simulink model "QEI_Polling"  (R2024b)
settings: Solver=FixedStepAuto  StartTime=0.0  StopTime=inf  FixedStep=0.001  RelTol=1e-3  EnableMultiTasking=on
libraries: stm32f4xxblockslib x5, stm32g4xxblockslib x3
settings Model: STM32="{\"DigitalPortRead\":[{\"ID\":\"untitled1:6\"},{\"ID\":\"untitled1:7\"},{\"ID\":\"untitled1:8\"},{\"ID\":\"untitled1:9\"},{\"ID\":\"untitled1:10\"},{\"ID\":\"QEI_Polling:10\"},{\"ID\":\"QEI_Polling:9\"},{\"ID\":\"QEI_Polling:8\"},{\"ID\":\"QEI_Polling:7\"},{\"ID\":\"QEI_Polling:6\"}],\"EncoderBlockForG4\":[{\"ID\":\"untitled1:29\"},{\"ID\":\"untitled1:30\"},{\"ID\":\"untitled1:31\"},{\"ID\":\"QEI_Polling:29\"},{\"ID\":\"QEI_Polling:30\"},{\"ID\":\"QEI_Polling:31\"}]}"  Creator=spwkp  LastModifiedBy=spwkp
settings OptimizationCC: DefaultParameterBehavior=Inlined  EnhancedBackFolding=on  PassReuseOutputArgsAs=Individual arguments  ZeroExternalMemoryAtStartup=off  ZeroInternalMemoryAtStartup=off  MaxStackSize=512  OptimizeBlockOrder=speed  DifferentSizesBufferReuse=on  OptimizationCustomize=off  EfficientTunableParamExpr=on
settings DebuggingCC: ParameterTunabilityLossMsg=error
settings HardwareCC: ProdBitPerPointer=32  ProdBitPerSizeT=32  ProdBitPerPtrDiffT=32  ProdLargestAtomicInteger=Long  ProdLargestAtomicFloat=Double  ProdWordSize=32  ProdLongLongMode=on  ProdHWDeviceType=ARM Compatible->ARM Cortex-M
settings SFSimCC: MATLABDynamicMemAlloc=off
settings RTWCC: Description=Embedded Coder  SystemTargetFile=ert.tlc  HardwareBoard=STM32G4xx Based  TemplateMakefile=ert_default_tmf  Toolchain=GNU Tools for ARM Embedded Processors
settings CodeAppCC: ForceParamTrailComments=on  IgnoreCustomStorageClasses=off  OperatorAnnotations=on  SimulinkDataObjDesc=on  SFDataObjDesc=on  InsertBlockDesc=on
settings ERTTargetCC: TargetLangStandard=C99 (ISO)  CodeReplacementLibrary=ARM Cortex-M  ExtModeTransport=3  ExtModeStaticAlloc=on  ExtModeStaticAllocSize=2048  ExtModeMexFile=ext_xcp  ExtModeIntrfLevel=Level2 - Open

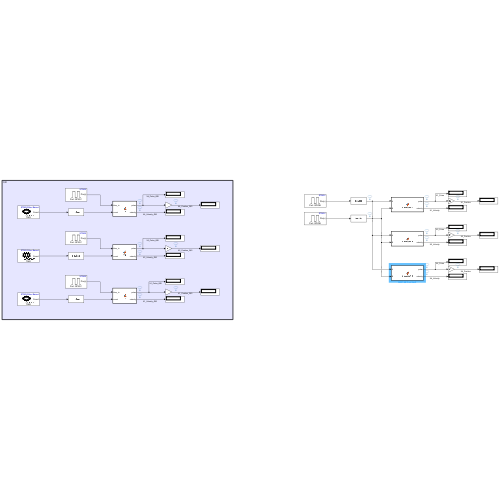
[thumbnail: Simulink's stored preview of the top-level diagram]
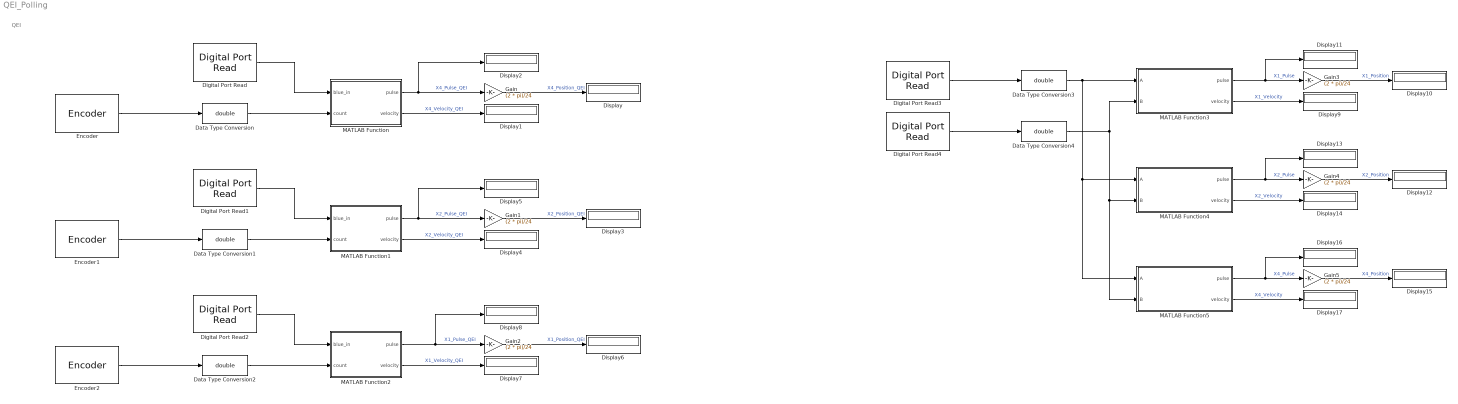
== system QEI_Polling ==
  note: QEI
  Data Type Conversion{,1..4} (5 alike) : DataTypeConversion  OutDataTypeStr=double  SaturateOnIntegerOverflow=off  RndMeth=Floor
  Digital Port Read : stm32f4xxblockslib/Digital Port Read  PortName=GPIOC  PinNumber=[13]  ReadOperation=on  IOAsArray=on  SampleTime=-1  EnableSimPort=off  hoistedMaskSrc=ECSoC/ECSimCodegen/Digital Port Read
      settings: LibrarySourceBlock=stm32g4xxblockslib/Digital Port Read
  Digital Port Read1 : stm32f4xxblockslib/Digital Port Read  PortName=GPIOC  PinNumber=[13]  ReadOperation=on  IOAsArray=on  SampleTime=-1  EnableSimPort=off  hoistedMaskSrc=ECSoC/ECSimCodegen/Digital Port Read
      settings: LibrarySourceBlock=stm32g4xxblockslib/Digital Port Read
  Digital Port Read2 : stm32f4xxblockslib/Digital Port Read  PortName=GPIOC  PinNumber=[13]  ReadOperation=on  IOAsArray=on  SampleTime=-1  EnableSimPort=off  hoistedMaskSrc=ECSoC/ECSimCodegen/Digital Port Read
      settings: LibrarySourceBlock=stm32g4xxblockslib/Digital Port Read
  Digital Port Read3 : stm32f4xxblockslib/Digital Port Read  PortName=GPIOB  PinNumber=[5]  ReadOperation=on  IOAsArray=on  SampleTime=-1  EnableSimPort=off  hoistedMaskSrc=ECSoC/ECSimCodegen/Digital Port Read
      settings: LibrarySourceBlock=stm32g4xxblockslib/Digital Port Read
  Digital Port Read4 : stm32f4xxblockslib/Digital Port Read  PortName=GPIOB  PinNumber=[4]  ReadOperation=on  IOAsArray=on  SampleTime=-1  EnableSimPort=off  hoistedMaskSrc=ECSoC/ECSimCodegen/Digital Port Read
      settings: LibrarySourceBlock=stm32g4xxblockslib/Digital Port Read
  Display{,1..17} (18 alike) : Display
  Encoder : stm32g4xxblockslib/Encoder  TimerModule=TIM3  EnableResetInput=off  OutputCountAfterFirstIndex=off  OutputValidIndex=off  OutputDirection=off  OutputStatus=off  SampleTime=-1
  Encoder1 : stm32g4xxblockslib/Encoder  TimerModule=TIM4  EnableResetInput=off  OutputCountAfterFirstIndex=off  OutputValidIndex=off  OutputDirection=off  OutputStatus=off  SampleTime=-1
  Encoder2 : stm32g4xxblockslib/Encoder  TimerModule=TIM8  EnableResetInput=off  OutputCountAfterFirstIndex=off  OutputValidIndex=off  OutputDirection=off  OutputStatus=off  SampleTime=-1
  Gain{,1..5} (6 alike) : Gain  Gain=(2 * pi)/24
  MATLAB Function : MATLAB Function  TreatAsAtomicUnit=on
  MATLAB Function1 : MATLAB Function  TreatAsAtomicUnit=on
  MATLAB Function2 : MATLAB Function  TreatAsAtomicUnit=on
  MATLAB Function3 : MATLAB Function  TreatAsAtomicUnit=on
  MATLAB Function4 : MATLAB Function  TreatAsAtomicUnit=on
  MATLAB Function5 : MATLAB Function  TreatAsAtomicUnit=on
  wires:
  Data Type Conversion/1 -> MATLAB Function/2(count)
  Encoder1/1 -> Data Type Conversion1/1
  Gain3/1 -> Display10/1  "X1_Position"
  MATLAB Function2/2(velocity) -> Display7/1  "X1_Velocity_QEI"
  MATLAB Function3/2(velocity) -> Display9/1  "X1_Velocity"
  Data Type Conversion3/1 -> MATLAB Function4/1(A), MATLAB Function5/1(A), MATLAB Function3/1(A)
  Data Type Conversion2/1 -> MATLAB Function2/2(count)
  MATLAB Function3/1(pulse) -> Display11/1, Gain3/1  "X1_Pulse"
  Digital Port Read1/1 -> MATLAB Function1/1(blue_in)
  Encoder2/1 -> Data Type Conversion2/1
  Digital Port Read/1 -> MATLAB Function/1(blue_in)
  Digital Port Read4/1 -> Data Type Conversion4/1
  MATLAB Function5/1(pulse) -> Display16/1, Gain5/1  "X4_Pulse"
  MATLAB Function/1(pulse) -> Display2/1, Gain/1  "X4_Pulse_QEI"
  Gain5/1 -> Display15/1  "X4_Position"
  Data Type Conversion1/1 -> MATLAB Function1/2(count)
  MATLAB Function1/2(velocity) -> Display4/1  "X2_Velocity_QEI"
  Data Type Conversion4/1 -> MATLAB Function4/2(B), MATLAB Function5/2(B), MATLAB Function3/2(B)
  Gain1/1 -> Display3/1  "X2_Position_QEI"
  Digital Port Read3/1 -> Data Type Conversion3/1
  MATLAB Function4/1(pulse) -> Display13/1, Gain4/1  "X2_Pulse"
  Encoder/1 -> Data Type Conversion/1
  Digital Port Read2/1 -> MATLAB Function2/1(blue_in)
  MATLAB Function5/2(velocity) -> Display17/1  "X4_Velocity"
  MATLAB Function1/1(pulse) -> Display5/1, Gain1/1  "X2_Pulse_QEI"
  Gain/1 -> Display/1  "X4_Position_QEI"
  MATLAB Function/2(velocity) -> Display1/1  "X4_Velocity_QEI"
  Gain4/1 -> Display12/1  "X2_Position"
  Gain2/1 -> Display6/1  "X1_Position_QEI"
  MATLAB Function4/2(velocity) -> Display14/1  "X2_Velocity"
  MATLAB Function2/1(pulse) -> Display8/1, Gain2/1  "X1_Pulse_QEI"

== matlab function QEI_Polling/MATLAB Function1 ==
  data: blue_in input; pulse output; count input; velocity output
function [pulse, velocity] = X4(blue_in, count)
    %#codegen
    
    % ประกาศตัวแปร persistent เพื่อเก็บค่าตัวนับก่อนหน้าและตำแหน่งที่คลายห่อก่อนหน้า
    persistent previousCount unwrappedPositionPrev;
    
    % กำหนดค่าเริ่มต้นให้ตัวแปร persistent เมื่อเรียกใช้งานครั้งแรก
    if isempty(previousCount)
        previousCount = count;
        unwrappedPositionPrev = 0;  % กำหนดตำแหน่งคลายห่อเริ่มต้นเป็นศูนย์
    end

    % กำหนดขอบเขตของ encoder
    encoderMax = 65520;   % ค่าสูงสุดสำหรับ encoder แบบ 16-bit (0-65535)
    threshold = encoderMax / 2;  % ค่า threshold สำหรับตรวจจับ overflow หรือ underflow

    % คำนวณค่าความแตกต่างระหว่างค่าปัจจุบันกับค่าก่อนหน้า
    diff_count = count - previousCount;

    % คำนวณความเร็วเชิงมุม (Angular Velocity)
    Ts = 0.01; % กำหนด Sampling Time (เช่น 10ms)
    PPR = 24; % จำนวนพัลส์ต่อรอบ
    velocity = ((diff_count / PPR) / Ts) * 60; % Velocity เป็น RPM

    % ตรวจจับการ overflow และ underflow
    if diff_count > threshold
        % พบการ overflow (เช่น count เปลี่ยนจาก 65535 กลับไปที่ 0)
        pulse = unwrappedPositionPrev + (diff_count - encoderMax);
    elseif diff_count < -threshold
        % พบการ underflow (เช่น count เปลี่ยนจาก 0 เป็น 65535)
        pulse = unwrappedPositionPrev + (diff_count + encoderMax);
    else
        % กรณีปกติที่ไม่มี overflow/underflow
        pulse = unwrappedPositionPrev + diff_count;
    end

    if blue_in == 1
        pulse = 0;
        velocity = 0;
    end
    % อัปเดตตัวแปร persistent เพื่อใช้ในรอบถัดไป
    previousCount = count;
    unwrappedPositionPrev = pulse; 
end

== matlab function QEI_Polling/MATLAB Function ==
  data: blue_in input; pulse output; count input; velocity output
function [pulse, velocity] = X4(blue_in, count)
    %#codegen
    
    % ประกาศตัวแปร persistent เพื่อเก็บค่าตัวนับก่อนหน้าและตำแหน่งที่คลายห่อก่อนหน้า
    persistent previousCount unwrappedPositionPrev;
    
    % กำหนดค่าเริ่มต้นให้ตัวแปร persistent เมื่อเรียกใช้งานครั้งแรก
    if isempty(previousCount)
        previousCount = count;
        unwrappedPositionPrev = 0;  % กำหนดตำแหน่งคลายห่อเริ่มต้นเป็นศูนย์
    end

    % กำหนดขอบเขตของ encoder
    encoderMax = 65520;   % ค่าสูงสุดสำหรับ encoder แบบ 16-bit (0-65535)
    threshold = encoderMax / 2;  % ค่า threshold สำหรับตรวจจับ overflow หรือ underflow

    % คำนวณค่าความแตกต่างระหว่างค่าปัจจุบันกับค่าก่อนหน้า
    diff_count = count - previousCount;

    % คำนวณความเร็วเชิงมุม (Angular Velocity)
    Ts = 0.01; % กำหนด Sampling Time (เช่น 10ms)
    PPR = 24; % จำนวนพัลส์ต่อรอบ
    velocity = ((diff_count / PPR) / Ts) * 60; % Velocity เป็น RPM

    % ตรวจจับการ overflow และ underflow
    if diff_count > threshold
        % พบการ overflow (เช่น count เปลี่ยนจาก 65535 กลับไปที่ 0)
        pulse = unwrappedPositionPrev + (diff_count - encoderMax);
    elseif diff_count < -threshold
        % พบการ underflow (เช่น count เปลี่ยนจาก 0 เป็น 65535)
        pulse = unwrappedPositionPrev + (diff_count + encoderMax);
    else
        % กรณีปกติที่ไม่มี overflow/underflow
        pulse = unwrappedPositionPrev + diff_count;
    end

    if blue_in == 1
        pulse = 0;
        velocity = 0;
    end
    % อัปเดตตัวแปร persistent เพื่อใช้ในรอบถัดไป
    previousCount = count;
    unwrappedPositionPrev = pulse; 
end

== matlab function QEI_Polling/MATLAB Function2 ==
  data: blue_in input; pulse output; count input; velocity output
function [pulse, velocity] = X1(blue_in, count)
    %#codegen
    
    % ประกาศตัวแปร persistent เพื่อเก็บค่าตัวนับก่อนหน้าและตำแหน่งที่คลายห่อก่อนหน้า
    persistent previousCount unwrappedPositionPrev;
    
    % กำหนดค่าเริ่มต้นให้ตัวแปร persistent เมื่อเรียกใช้งานครั้งแรก
    if isempty(previousCount)
        previousCount = count;
        unwrappedPositionPrev = 0;  % กำหนดตำแหน่งคลายห่อเริ่มต้นเป็นศูนย์
    end

    % กำหนดขอบเขตของ encoder
    encoderMax = 65520;   % ค่าสูงสุดสำหรับ encoder แบบ 16-bit (0-65535)
    threshold = encoderMax / 2;  % ค่า threshold สำหรับตรวจจับ overflow หรือ underflow

    % คำนวณค่าความแตกต่างระหว่างค่าปัจจุบันกับค่าก่อนหน้า
    diff_count = count - previousCount;

    % คำนวณความเร็วเชิงมุม (Angular Velocity)
    Ts = 0.01; % กำหนด Sampling Time (เช่น 10ms)
    PPR = 24; % จำนวนพัลส์ต่อรอบ
    velocity = ((diff_count / PPR) / Ts) * 60; % Velocity เป็น RPM

    % ตรวจจับการ overflow และ underflow
    if diff_count > threshold
        % พบการ overflow (เช่น count เปลี่ยนจาก 65535 กลับไปที่ 0)
        pulse = unwrappedPositionPrev + (diff_count - encoderMax);
    elseif diff_count < -threshold
        % พบการ underflow (เช่น count เปลี่ยนจาก 0 เป็น 65535)
        pulse = unwrappedPositionPrev + (diff_count + encoderMax);
    else
        % กรณีปกติที่ไม่มี overflow/underflow
        pulse = unwrappedPositionPrev + diff_count;
    end

    if blue_in == 1
        pulse = 0;
        velocity = 0;
    end
    % อัปเดตตัวแปร persistent เพื่อใช้ในรอบถัดไป
    previousCount = count;
    unwrappedPositionPrev = pulse; 
end

== matlab function QEI_Polling/MATLAB Function3 ==
  data: A input double size=[1 1]; pulse output; B input double size=[1 1]; velocity output
function [pulse, velocity] = EncoderX1(A, B)
   
    persistent lastA count lastCount;
    if isempty(lastA) || isempty(count) || isempty(lastCount)
        lastA = 0;
        count = 0;
        lastCount = 0;
    end
    
    currentA = A;  
    currentB = B;  
    
    if lastA ~= currentA
        if currentB == 1 && currentA == 1
            count = count - 1; 
        elseif currentB == 0 && currentA == 1
            count = count + 1;  
        end
    end
    
    velocity = ((count - lastCount) / 0.001) * 60;
    
    lastA = currentA;
    lastCount = count;
    
    pulse = count;
end

== matlab function QEI_Polling/MATLAB Function4 ==
  data: A input double size=[1 1]; pulse output; B input double size=[1 1]; velocity output
function [pulse, velocity] = EncoderX2(A, B)
   
    persistent lastA count lastCount;
    if isempty(lastA) || isempty(count) || isempty(lastCount)
        lastA = 0;
        count = 0;
        lastCount = 0;
    end
    
    currentA = A;  
    currentB = B;  
    
    if lastA ~= currentA
        if currentB == 1 && currentA == 1 && lastA == 0
            count = count - 1;  % Forward count
        elseif currentB == 0 && currentA == 1 && lastA == 0
            count = count + 1;  % Backward count
        elseif currentB == 1 && currentA == 0 && lastA == 1
            count = count + 1;
        elseif currentB == 0 && currentA == 0 && lastA == 1
            count = count - 1;
        end
    end
    
    velocity = ((count - lastCount) / 0.001) * 60;
    
    lastA = currentA;
    lastCount = count;
    
    pulse = count;
end

== matlab function QEI_Polling/MATLAB Function5 ==
  data: A input double size=[1 1]; pulse output; B input double size=[1 1]; velocity output
function [pulse, velocity] = EncoderX4(A, B)

    persistent lastA lastB count lastCount;

    if isempty(lastA) || isempty(lastB) || isempty(count) || isempty(lastCount)
        lastA = 0;
        lastB = 0;
        count = 0;
        lastCount = 0;
    end
    
    
    if lastA == 0 && A == 1
        if B  == 0
            count = count + 1;
        else
            count = count - 1;
        end
    elseif lastA == 1 && A == 0
        if B == 0
            count = count - 1;
        else
            count = count + 1;
        end
    elseif lastB == 0 && B == 1
        if A == 0
            count = count + 1;
        else
            count = count - 1;
        end
    elseif lastB == 1 && B == 0
        if A == 0
            count = count - 1;
        else
            count = count + 1;
        end
    end
        
    
    velocity = ((count - lastCount) / 0.001) * 60;
    
    lastA = A;
    lastB = B;
    lastCount = count;
    
    pulse = count;
end
